simulink library "lib_accessory2"  (Simulink 4.1.1)
values from neighbouring files (symbols this model uses):
  logFlag = 1    [advSACompMaskInit.m]    (also in advSACompMaskInitR13.m)
undefined symbols (not defined in the file or in its folder): acc_abc_dutycycle, acc_abc_init, acc_ac_dutycycle, acc_ac_init, acc_acdc_inverter_eff, acc_alt_init, acc_dcdc_eff, acc_ef_dutycycle, acc_ef_init, acc_elec_eff, acc_elec_efficiency, acc_elec_pwr, acc_mech_eff, acc_mech_pwr, acc_mech_trq, acc_op_dutycycle, acc_op_init, acc_ps_dutycycle, acc_ps_init, acc_sindafile, acc_wp_dutycycle, acc_wp_init, amb_tmp, ess_on, fc_on, generalName, map_spd, max_pwr, tc_gc_to_fc_ratio, time_step, vc_idle_bool, vc_idle_spd, vinf
libraries: lib_cosimulation x29, lib_accessory2 x15, lib_outputs x11, simulink3 x10, lib_accessory x8, lib_etc x2
(part 2 of 5)

== system lib_accessory2/Elec Aux Loads 14V Pwr/Engine ==
  Average Watts : Constant  Value=vinf.AuxLoads.Engine.AverageWatts
  Memory : Memory  X0=0  InheritSampleTime=off
      settings: RTWStateStorageClass=Auto
  On : Constant  Value=vinf.AuxLoads.Engine.On
  Product : Product  Inputs=4  Multiplication=Element-wise(.*)  SaturateOnIntegerOverflow=on
  Out1 : Outport  Port=1
  wires:
  Memory/1 -> Product/2
  [engine_on] -> Memory/1
  [key_on] -> Product/3
  On/1 -> Product/1
  Product/1 -> Out1/1
  Average Watts/1 -> Product/4

== system lib_accessory2/Elec Aux Loads 14V Pwr/ExternalLights ==
  Average Watts : Constant  Value=vinf.AuxLoads.ExternalLights.AverageWatts
  On : Constant  Value=vinf.AuxLoads.ExternalLights.On
  Product : Product  Inputs=3  Multiplication=Element-wise(.*)  SaturateOnIntegerOverflow=on
  Subsystem : lib_cosimulation/Subsystem  ModelName='ExternalLights'
  Out1 : Outport  Port=1
  wires:
  Average Watts/1 -> Product/3
  On/1 -> Product/1
  Subsystem/1 -> Product/2
  Product/1 -> Out1/1

== system lib_accessory2/Elec Aux Loads 14V Pwr/FrontHVAC ==
  Average Watts : Constant  Value=vinf.AuxLoads.FrontHVAC.AverageWatts
  On : Constant  Value=vinf.AuxLoads.FrontHVAC.On
  Product : Product  Inputs=3  Multiplication=Element-wise(.*)  SaturateOnIntegerOverflow=on
  Subsystem : lib_cosimulation/Subsystem  ModelName='FrontHVAC'
  Out1 : Outport  Port=1
  wires:
  Average Watts/1 -> Product/3
  On/1 -> Product/1
  Subsystem/1 -> Product/2
  Product/1 -> Out1/1

== system lib_accessory2/Elec Aux Loads 14V Pwr/FrontWipers ==
  Average Watts : Constant  Value=vinf.AuxLoads.FrontWipers.AverageWatts
  On : Constant  Value=vinf.AuxLoads.FrontWipers.On
  Product : Product  Inputs=3  Multiplication=Element-wise(.*)  SaturateOnIntegerOverflow=on
  Subsystem : lib_cosimulation/Subsystem  ModelName='FrontWipers'
  Out1 : Outport  Port=1
  wires:
  Average Watts/1 -> Product/3
  On/1 -> Product/1
  Subsystem/1 -> Product/2
  Product/1 -> Out1/1

== system lib_accessory2/Elec Aux Loads 14V Pwr/HeatedSeats ==
  Average Watts : Constant  Value=vinf.AuxLoads.HeatedSeats.AverageWatts
  Num : Constant  Value=vinf.AuxLoads.HeatedSeats.Num
  On : Constant  Value=vinf.AuxLoads.HeatedSeats.On
  Product : Product  Inputs=4  Multiplication=Element-wise(.*)  SaturateOnIntegerOverflow=on
  Subsystem : lib_cosimulation/Subsystem  ModelName='HeatedSeats'
  Out1 : Outport  Port=1
  wires:
  Subsystem/1 -> Product/3
  Product/1 -> Out1/1
  Average Watts/1 -> Product/4
  On/1 -> Product/1
  Num/1 -> Product/2

== system lib_accessory2/Elec Aux Loads 14V Pwr/Misc ==
  Average Watts : Constant  Value=vinf.AuxLoads.Misc.AverageWatts
  On : Constant  Value=vinf.AuxLoads.Misc.On
  Product : Product  Inputs=3  Multiplication=Element-wise(.*)  SaturateOnIntegerOverflow=on
  Out1 : Outport  Port=1
  wires:
  Average Watts/1 -> Product/3
  [key_on] -> Product/2
  On/1 -> Product/1
  Product/1 -> Out1/1

== system lib_accessory2/Elec Aux Loads 14V Pwr/RadiatorCoolingFan ==
  Average Watts : Constant  Value=vinf.AuxLoads.RadiatorCoolingFan.AverageWatts
  On : Constant  Value=vinf.AuxLoads.RadiatorCoolingFan.On
  Product : Product  Inputs=3  Multiplication=Element-wise(.*)  SaturateOnIntegerOverflow=on
  Subsystem : lib_cosimulation/Subsystem  ModelName='RadiatorCoolingFan'
  Out1 : Outport  Port=1
  wires:
  Average Watts/1 -> Product/3
  On/1 -> Product/1
  Subsystem/1 -> Product/2
  Product/1 -> Out1/1

== system lib_accessory2/Elec Aux Loads 14V Pwr/Radio ==
  Average Watts : Constant  Value=vinf.AuxLoads.Radio.AverageWatts
  Num : Constant  Value=vinf.AuxLoads.Radio.Num
  On : Constant  Value=vinf.AuxLoads.Radio.On
  Product : Product  Inputs=4  Multiplication=Element-wise(.*)  SaturateOnIntegerOverflow=on
  Subsystem : lib_cosimulation/Subsystem  ModelName='Radio'
  Out1 : Outport  Port=1
  wires:
  Subsystem/1 -> Product/3
  Average Watts/1 -> Product/4
  On/1 -> Product/1
  Num/1 -> Product/2
  Product/1 -> Out1/1

== system lib_accessory2/Elec Aux Loads 14V Pwr/RearDefrost ==
  Average Watts : Constant  Value=vinf.AuxLoads.RearDefrost.AverageWatts
  On : Constant  Value=vinf.AuxLoads.RearDefrost.On
  Product : Product  Inputs=3  Multiplication=Element-wise(.*)  SaturateOnIntegerOverflow=on
  Subsystem : lib_cosimulation/Subsystem  ModelName='RearDefrost'
  Out1 : Outport  Port=1
  wires:
  Subsystem/1 -> Product/2
  Average Watts/1 -> Product/3
  On/1 -> Product/1
  Product/1 -> Out1/1

== system lib_accessory2/Elec Aux Loads 14V Pwr/RearHVAC ==
  Average Watts : Constant  Value=vinf.AuxLoads.RearHVAC.AverageWatts
  On : Constant  Value=vinf.AuxLoads.RearHVAC.On
  Product : Product  Inputs=3  Multiplication=Element-wise(.*)  SaturateOnIntegerOverflow=on
  Subsystem : lib_cosimulation/Subsystem  ModelName='RearHVAC'
  Out1 : Outport  Port=1
  wires:
  Average Watts/1 -> Product/3
  On/1 -> Product/1
  Subsystem/1 -> Product/2
  Product/1 -> Out1/1

== system lib_accessory2/Elec Aux Loads 14V Pwr/RearWipers ==
  Average Watts : Constant  Value=vinf.AuxLoads.RearWipers.AverageWatts
  On : Constant  Value=vinf.AuxLoads.RearWipers.On
  Product : Product  Inputs=3  Multiplication=Element-wise(.*)  SaturateOnIntegerOverflow=on
  Subsystem : lib_cosimulation/Subsystem  ModelName='RearWipers'
  Out1 : Outport  Port=1
  wires:
  Average Watts/1 -> Product/3
  On/1 -> Product/1
  Subsystem/1 -> Product/2
  Product/1 -> Out1/1

== system lib_accessory2/Elec Aux Loads 14V Pwr/Starter ==
  Product1 : Product  Inputs=2  Multiplication=Element-wise(.*)  SaturateOnIntegerOverflow=on
  Starter : lib_cosimulation/14V Load Control/Starter
      settings: RTWFcnNameOpts=Auto  RTWFileNameOpts=Auto
  starter_load (power) : Constant  Value=vinf.AuxLoads.Starter.AverageWatts
  Out1 : Outport  Port=1
  wires:
  Starter/1 -> Product1/1
  starter_load (power)/1 -> Product1/2
  Product1/1 -> Out1/1

== system lib_accessory2/Elec Aux Loads 14V Pwr/TurnSignals ==
  Average Watts : Constant  Value=vinf.AuxLoads.TurnSignals.AverageWatts
  On : Constant  Value=vinf.AuxLoads.TurnSignals.On
  Product : Product  Inputs=3  Multiplication=Element-wise(.*)  SaturateOnIntegerOverflow=on
  Subsystem : lib_cosimulation/Subsystem  ModelName='TurnSignals'
  Out1 : Outport  Port=1
  wires:
  Average Watts/1 -> Product/3
  On/1 -> Product/1
  Subsystem/1 -> Product/2
  Product/1 -> Out1/1

== system lib_accessory2/Elec Aux Loads HiV Pwr/CurrentLoad1 ==
  Average Watts : Constant  Value=vinf.AuxLoads.CurrentLoad1.AverageWatts
  On : Constant  Value=vinf.AuxLoads.CurrentLoad1.On
  Product : Product  Inputs=3  Multiplication=Element-wise(.*)  SaturateOnIntegerOverflow=on
  Subsystem : lib_cosimulation/Subsystem  ModelName='CurrentLoad1'
  Out1 : Outport  Port=1
  wires:
  Product/1 -> Out1/1
  Subsystem/1 -> Product/2
  On/1 -> Product/1
  Average Watts/1 -> Product/3

== system lib_accessory2/Elec Aux Loads HiV Pwr/PowerLoad1 ==
  Average Watts : Constant  Value=vinf.AuxLoads.PowerLoad1.AverageWatts
  On : Constant  Value=vinf.AuxLoads.PowerLoad1.On
  Product : Product  Inputs=3  Multiplication=Element-wise(.*)  SaturateOnIntegerOverflow=on
  Subsystem : lib_cosimulation/Subsystem  ModelName='PowerLoad1'
  Out1 : Outport  Port=1
  wires:
  Product/1 -> Out1/1
  On/1 -> Product/1
  Average Watts/1 -> Product/3
  Subsystem/1 -> Product/2

== system lib_accessory2/Elec Aux Loads HiV Pwr/PowerLoad2 ==
  Average Watts : Constant  Value=vinf.AuxLoads.PowerLoad2.AverageWatts
  On : Constant  Value=vinf.AuxLoads.PowerLoad2.On
  Product : Product  Inputs=3  Multiplication=Element-wise(.*)  SaturateOnIntegerOverflow=on
  Subsystem : lib_cosimulation/Subsystem  ModelName='PowerLoad2'
  Out1 : Outport  Port=1
  wires:
  Subsystem/1 -> Product/2
  Average Watts/1 -> Product/3
  On/1 -> Product/1
  Product/1 -> Out1/1

== system lib_accessory2/Elec Aux Loads HiV Pwr/PowerLoad3 ==
  Average Watts : Constant  Value=vinf.AuxLoads.PowerLoad3.AverageWatts
  On : Constant  Value=vinf.AuxLoads.PowerLoad3.On
  Product : Product  Inputs=3  Multiplication=Element-wise(.*)  SaturateOnIntegerOverflow=on
  Subsystem : lib_cosimulation/Subsystem  ModelName='PowerLoad3'
  Out1 : Outport  Port=1
  wires:
  Product/1 -> Out1/1
  On/1 -> Product/1
  Average Watts/1 -> Product/3
  Subsystem/1 -> Product/2

== system lib_accessory2/Elec Aux Loads HiV Pwr/SpeedLoad1 ==
  On : Constant  Value=vinf.AuxLoads.SpeedLoad1.On
  Product : Product  Inputs=3  Multiplication=Element-wise(.*)  SaturateOnIntegerOverflow=on
  Subsystem : lib_cosimulation/Subsystem  ModelName='SpeedLoad1'
  "rad/s -> rpm1" : Gain  Gain=60/(2*pi)  Multiplication=Element-wise(K.*u)  SaturateOnIntegerOverflow=on
  speed (rpm) vs load (watts) : Lookup  InputValues=[vinf.AuxLoads.SpeedLoad1.Data(1,1),vinf.AuxLoads.SpeedLoad1.Data(2,1)]  OutputValues=[vinf.AuxLoads.SpeedLoad1.Data(1,2),vinf.AuxLoads.SpeedLoad1.Data(2,2)]
  Out1 : Outport  Port=1
  wires:
  Product/1 -> Out1/1
  Subsystem/1 -> Product/2
  On/1 -> Product/1
  speed (rpm) vs load (watts)/1 -> Product/3
  [w_APU_speed] -> "rad/s -> rpm1"/1
  "rad/s -> rpm1"/1 -> speed (rpm) vs load (watts)/1

== system lib_accessory2/Elec Aux Loads HiV Pwr/Starter ==
  Product1 : Product  Inputs=2  Multiplication=Element-wise(.*)  SaturateOnIntegerOverflow=on
  Starter : Subsystem
      settings: RTWFcnNameOpts=Auto  RTWFileNameOpts=Auto
  starter_load (power) : Constant  Value=vinf.AuxLoads.Starter.AverageWatts
  Out1 : Outport  Port=1
  wires:
  Product1/1 -> Out1/1
  starter_load (power)/1 -> Product1/2
  Starter/1(Starter_OnOff_Control) -> Product1/1

== system lib_accessory2/SubLibraries/Shaft Speed and Actual Load Auxiliary Device ==
  angular  speed of engine  shaft (rad/s) : Inport  Port=1  LatchInput=off
  load on device (W) : Inport  Port=2  LatchInput=off
  Gain : Gain  Gain=1/conv_eff  Multiplication=Element-wise(K.*u)  SaturateOnIntegerOverflow=on
  Mux : Mux  Inputs=2
  device power requirements : MATLABFcn  MATLABFcn=feval(pwr_func, u(1), u(2))  OutputDimensions=1  OutputSignalType=real  Output1D=on
  powr required by device (W) : Outport  Port=1
  wires:
  angular  speed of engine  shaft (rad/s)/1 -> Mux/1
  Gain/1 -> Mux/2
  load on device (W)/1 -> Gain/1
  device power requirements/1 -> powr required by device (W)/1
  Mux/1 -> device power requirements/1

== system lib_accessory2/SubLibraries/Shaft Speed and Actual Load Auxiliary Device--lookuptable ==
  angular  speed of engine  shaft (rad/s) : Inport  Port=1  LatchInput=off
  load on device (W) : Inport  Port=2  LatchInput=off
  Constant : Constant  Value=0.0
  Constant1 : Constant  Value=eps
  Gain : Gain  Gain=1/conv_eff  Multiplication=Element-wise(K.*u)  SaturateOnIntegerOverflow=on
  Look-Up Table : Lookup  InputValues=map_spd  OutputValues=max_pwr
  Look-Up Table (2-D) : simulink3/Functions & Tables/Look-Up Table (2-D)  x=map_spd  y=map_load  t=pwr_map
  Product : Product  Inputs=*/  Multiplication=Element-wise(.*)  SaturateOnIntegerOverflow=on
  Relational Operator : RelationalOperator  Operator=~=
  Saturation : Saturate  UpperLimit=1.0  LowerLimit=0.0  LinearizeAsGain=on
  Saturation1 : Saturate  UpperLimit=maxSpd  LowerLimit=minSpd  LinearizeAsGain=on
  Switch : Switch  Threshold=0.5
  powr required by device (W) : Outport  Port=1
  wires:
  load on device (W)/1 -> Gain/1
  Look-Up Table (2-D)/1 -> powr required by device (W)/1
  angular  speed of engine  shaft (rad/s)/1 -> Saturation1/1
  [spd] -> Look-Up Table (2-D)/1
  Saturation1/1 -> [spd]
  Gain/1 -> Product/1
  [spd] -> Look-Up Table/1
  Product/1 -> Saturation/1
  Saturation/1 -> Look-Up Table (2-D)/2
  Look-Up Table/1 -> Relational Operator/1, Switch/1
  Constant/1 -> Relational Operator/2
  Relational Operator/1 -> Switch/2
  Constant1/1 -> Switch/3
  Switch/1 -> Product/2

== system lib_accessory2/SubLibraries/Shaft Speed and Time Loaded Auxiliary Device ==
  angular  speed of engine  shaft (rad/s) : Inport  Port=1  LatchInput=off
  elapsed time since start of simulation (s) : Inport  Port=2  LatchInput=off
  Mux : Mux  Inputs=2
  Sat : Saturate  UpperLimit=1.0  LowerLimit=0.0  LinearizeAsGain=on
  device duty  schedule by time : Subsystem  mask(Repeating table){t=acc_duty(:,1), y=acc_duty(:,2)}
      mask prompts: t "Input values:"; y "Output values:"
      mask help:
      | Repeating table.
      | Enter values of input and output for first cycle.
      mask init:
      | period = max(@1);
      settings: RTWFcnNameOpts=Auto  RTWFileNameOpts=Auto
      mask Help: Repeats cycle given in table. Input values should be monotonically increasing.
  device power requirements : MATLABFcn  MATLABFcn=feval(pwr_func, u(1), u(2))  OutputDimensions=1  OutputSignalType=real  Output1D=on
  powr required by device (W) : Outport  Port=1
  "duty cycle (1=\"on full power\" & 0=\"off\")" : Outport  Port=2
  wires:
  Mux/1 -> device power requirements/1
  angular  speed of engine  shaft (rad/s)/1 -> Mux/1
  device power requirements/1 -> powr required by device (W)/1
  elapsed time since start of simulation (s)/1 -> device duty  schedule by time/1(distance travelled (m))
  device duty  schedule by time/1(out_1) -> Sat/1
  Sat/1 -> Mux/2, "duty cycle (1=\"on full power\" & 0=\"off\")"/1

== system lib_accessory2/SubLibraries/Shaft Speed and Time Loaded Auxiliary Device--lookuptable ==
  angular  speed of engine  shaft (rad/s) : Inport  Port=1  LatchInput=off
  elapsed time since start of simulation (s) : Inport  Port=2  LatchInput=off
  Look-Up Table (2-D) : simulink3/Functions & Tables/Look-Up Table (2-D)  x=map_spd  y=map_load  t=pwr_map
  Sat : Saturate  UpperLimit=1.0  LowerLimit=0.0  LinearizeAsGain=on
  Sat1 : Saturate  UpperLimit=maxSpd  LowerLimit=minSpd  LinearizeAsGain=on
  device duty  schedule by time : Subsystem  mask(Repeating table){t=acc_duty(:,1), y=acc_duty(:,2)}
      mask prompts: t "Input values:"; y "Output values:"
      mask help:
      | Repeating table.
      | Enter values of input and output for first cycle.
      mask init:
      | period = max(@1);
      settings: RTWFcnNameOpts=Auto  RTWFileNameOpts=Auto
      mask Help: Repeats cycle given in table. Input values should be monotonically increasing.
  powr required by device (W) : Outport  Port=1
  "duty cycle (1=\"on full power\" & 0=\"off\")" : Outport  Port=2
  wires:
  Look-Up Table (2-D)/1 -> powr required by device (W)/1
  elapsed time since start of simulation (s)/1 -> device duty  schedule by time/1(distance travelled (m))
  device duty  schedule by time/1(out_1) -> Sat/1
  Sat/1 -> "duty cycle (1=\"on full power\" & 0=\"off\")"/1, Look-Up Table (2-D)/2
  angular  speed of engine  shaft (rad/s)/1 -> Sat1/1
  Sat1/1 -> Look-Up Table (2-D)/1

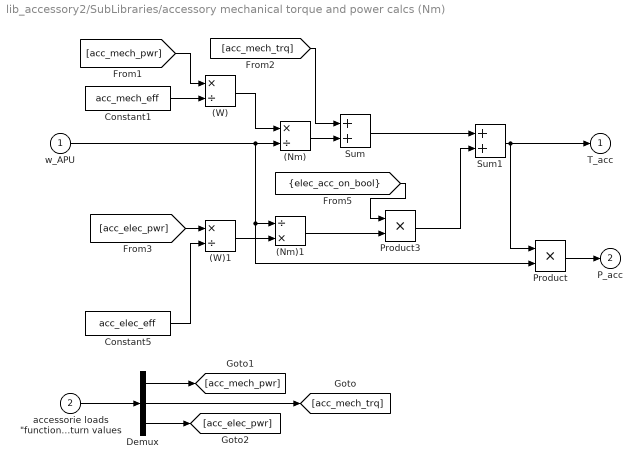
== system lib_accessory2/SubLibraries/accessory mechanical torque and power calcs (Nm) ==
  w_APU : Inport  Port=1  LatchInput=off
  "accessorie loads \"function\" return values" : Inport  Port=2  LatchInput=off
  (Nm) : Product  Inputs=*/  Multiplication=Element-wise(.*)  SaturateOnIntegerOverflow=on
  (Nm)1 : Product  Inputs=/*  Multiplication=Element-wise(.*)  SaturateOnIntegerOverflow=on
  (W) : Product  Inputs=*/  Multiplication=Element-wise(.*)  SaturateOnIntegerOverflow=on
  (W)1 : Product  Inputs=*/  Multiplication=Element-wise(.*)  SaturateOnIntegerOverflow=on
  Constant1 : Constant  Value=acc_mech_eff
  Constant5 : Constant  Value=acc_elec_eff
  Demux : Demux  Outputs=3  BusSelectionMode=off
  Product : Product  Inputs=2  Multiplication=Element-wise(.*)  SaturateOnIntegerOverflow=on
  Product3 : Product  Inputs=2  Multiplication=Element-wise(.*)  SaturateOnIntegerOverflow=on
  Sum : Sum  Inputs=++  SaturateOnIntegerOverflow=on
  Sum1 : Sum  Inputs=++  SaturateOnIntegerOverflow=on
  T_acc : Outport  Port=1  InitialOutput=0
  P_acc : Outport  Port=2  InitialOutput=0
  wires:
  "accessorie loads \"function\" return values"/1 -> Demux/1
  Demux/3 -> [acc_elec_pwr]
  Demux/1 -> [acc_mech_pwr]
  Demux/2 -> [acc_mech_trq]
  Product/1 -> P_acc/1
  (W)/1 -> (Nm)/1
  Constant1/1 -> (W)/2
  [acc_mech_pwr] -> (W)/1
  (Nm)/1 -> Sum/2
  Sum/1 -> Sum1/1
  Sum1/1 -> Product/1, T_acc/1
  Constant5/1 -> (W)1/2
  (W)1/1 -> (Nm)1/2
  (Nm)1/1 -> Product3/2
  Product3/1 -> Sum1/2
  [elec_acc_on_bool] -> Product3/1
  [acc_mech_trq] -> Sum/1
  w_APU/1 -> (Nm)1/1, Product/2, (Nm)/2
  [acc_elec_pwr] -> (W)1/1

== system lib_accessory2/SubLibraries/data logging probes dummy ==
  In1 : Inport  Port=1  LatchInput=off
  Terminator : Terminator
  wires:
  In1/1 -> Terminator/1

== system lib_accessory2/SubLibraries/data logging probes for conventional mechanical loads ==
  In1 : Inport  Port=1  LatchInput=off
  Demux : Demux  Outputs=12  BusSelectionMode=off
  To Workspace : ToWorkspace  VariableName=acc_ac_pwr_out_a  SampleTime=-1  SaveFormat=Array
  To Workspace1 : ToWorkspace  VariableName=acc_pwr_steer_pwr_out_a  SampleTime=-1  SaveFormat=Array
  To Workspace10 : ToWorkspace  VariableName=acc_op_pwr_out_a  SampleTime=-1  SaveFormat=Array
  To Workspace11 : ToWorkspace  VariableName=acc_op_duty  SampleTime=-1  SaveFormat=Array
  To Workspace2 : ToWorkspace  VariableName=acc_air_comp_pwr_out_a  SampleTime=-1  SaveFormat=Array
  To Workspace3 : ToWorkspace  VariableName=acc_eng_fan_pwr_out_a  SampleTime=-1  SaveFormat=Array
  To Workspace4 : ToWorkspace  VariableName=acc_alt_pwr_out_a  SampleTime=-1  SaveFormat=Array
  To Workspace5 : ToWorkspace  VariableName=acc_14elec_pwr_out_a  SampleTime=-1  SaveFormat=Array
  To Workspace6 : ToWorkspace  VariableName=acc_ps_duty  SampleTime=-1  SaveFormat=Array
  To Workspace7 : ToWorkspace  VariableName=acc_air_comp_duty  SampleTime=-1  SaveFormat=Array
  To Workspace8 : ToWorkspace  VariableName=acc_fan_duty  SampleTime=-1  SaveFormat=Array
  To Workspace9 : ToWorkspace  VariableName=acc_ac_duty  SampleTime=-1  SaveFormat=Array
  wires:
  Demux/12 -> To Workspace11/1
  Demux/11 -> To Workspace10/1
  Demux/10 -> To Workspace9/1
  Demux/9 -> To Workspace8/1
  Demux/8 -> To Workspace7/1
  Demux/7 -> To Workspace6/1
  Demux/6 -> To Workspace5/1
  Demux/5 -> To Workspace4/1
  Demux/4 -> To Workspace3/1
  Demux/3 -> To Workspace2/1
  Demux/2 -> To Workspace1/1
  Demux/1 -> To Workspace/1
  In1/1 -> Demux/1

== system lib_accessory2/SubLibraries/data probes ==
  In1 : Inport  Port=1  LatchInput=off
  data logging probes for conventional mechanical loads : lib_accessory/SubLibraries/data logging probes for conventional mechanical loads
      settings: RTWFcnNameOpts=Auto  RTWFileNameOpts=Auto
  wires:
  In1/1 -> data logging probes for conventional mechanical loads/1

== system lib_accessory2/SubLibraries/electrical power logging ==
  In1 : Inport  Port=1  LatchInput=off
  Gain : Gain  Gain=acc_elec_eff  Multiplication=Element-wise(K.*u)  SaturateOnIntegerOverflow=on
  enhancedToWorkspace : Subsystem  TreatAsAtomicUnit=on  mask(enhancedToWorkspace){generalName=generalName, specificName=elec_pwr_out_a, logFlag=logFlag}
      mask prompts: generalName "General Name [char-evaluated]"; specificName "Specific Name [char-literal]"; logFlag "Enable flag (1=on,0=off)"
      mask help: A wrapper for the Simulink "To Workspace" block that allows you to evaluate the name of the variable to log to workspace. This is useful to avoid the double logging errors that occur when you pull in two library models that attempt to log to the same variable.
      mask init:
      | enhancedToWsMaker
      settings: CopyFcn=breakLinkCopyFcn  ParentCloseFcn=breakLinkParCloseFcn  RTWFcnNameOpts=Auto  RTWFileNameOpts=Auto
      mask Help:
      | <h2>Enhanced To Workspace Block</h2>
      | <h3>Parameters</h3>
      | <UL>
      | <li><b>General Name:</b> This is the more general name of the variable. Variables are saved to the workspace as <i>generalName_specificName</i>. Note that this is an evaluated variable. If you would like to type in the value directly, it must be surrounded with single quotes. Otherwise you can input the name of a variable containing a char string.</li>
      | <li><b>Specific Name:</b> This is the specific name of the variable. Note that this is input as a char literal (i.e., you don't need quotes).</li>
      | <li><b>Enable Flag:</b> This flag should have the value of 0 or 1. If 0, the variable will not be logged to the workspace. If 1, the variable will be logged. This is done so that variable logging can be turned off to improve speed.</li>
      | </ul>
      | <h3>Overview</h3>
      | <p>The enhanced to workspace block was put together to allow one to dynamically resolve variable names at run time in simulink. This is most powerful when used in conjunction with a masked subsystem to allow multiple instances of that masked subsytem to be used in the same model. The strategy is to set the generalName in the block mask which will allow the block to change the general name for all variable logging on the fly.
      | <h3>Helper Files</h3>
      | <p>Three m-files are required by the enhancedToWorkspace block. These files are located in the &lt; ADVISOR root &gt;/GUI directory :
      | <ul>
      | <li><i>enhancedToWsMaker.m</i> This file runs the mask initialization for the block</li>
      | <li><i>breakLinkCopyFcn.m</i> This file is used by the block callback when the simulink block is copied. It is necessary to break the link to the enhancedToWorkspace similar to the To Workspace block in order for it to be able to configure itself. (Try copying simulink's To Workspace block--it is impossible to make a link)</li>
      | <li><i>breakLinkParCloseFcn.m</i> This file is similar to the breakLinkCopyFcn and is used when a parent system is closed</li>
      | </ul>
      | <hr>
      | 
      | <p>Created 2003-Jan-21, Michael Patrick O'Keefe, NREL</p>
      | 
      | <!--
      | <VARDEF>
      | <H3>var_name</H3>
      | <UL>
      | <LI><B>data type</B> data type here</LI>
      | <LI><B>units</B> units here</LI>
      | <LI><B>vehicle type</B> vehicle type here</LI>
      | <LI><B>description</B> description here</LI>
      | </UL>
      | </VARDEF>
      | -->
      mask Display: disp([generalName,'_',specificName])
  enhancedToWorkspace1 : Subsystem  TreatAsAtomicUnit=on  mask(enhancedToWorkspace){generalName=generalName, specificName=elec_pwr_in_a, logFlag=logFlag}
      mask prompts: generalName "General Name [char-evaluated]"; specificName "Specific Name [char-literal]"; logFlag "Enable flag (1=on,0=off)"
      mask help: A wrapper for the Simulink "To Workspace" block that allows you to evaluate the name of the variable to log to workspace. This is useful to avoid the double logging errors that occur when you pull in two library models that attempt to log to the same variable.
      mask init:
      | enhancedToWsMaker
      settings: CopyFcn=breakLinkCopyFcn  ParentCloseFcn=breakLinkParCloseFcn  RTWFcnNameOpts=Auto  RTWFileNameOpts=Auto
      mask Help:
      | <h2>Enhanced To Workspace Block</h2>
      | <h3>Parameters</h3>
      | <UL>
      | <li><b>General Name:</b> This is the more general name of the variable. Variables are saved to the workspace as <i>generalName_specificName</i>. Note that this is an evaluated variable. If you would like to type in the value directly, it must be surrounded with single quotes. Otherwise you can input the name of a variable containing a char string.</li>
      | <li><b>Specific Name:</b> This is the specific name of the variable. Note that this is input as a char literal (i.e., you don't need quotes).</li>
      | <li><b>Enable Flag:</b> This flag should have the value of 0 or 1. If 0, the variable will not be logged to the workspace. If 1, the variable will be logged. This is done so that variable logging can be turned off to improve speed.</li>
      | </ul>
      | <h3>Overview</h3>
      | <p>The enhanced to workspace block was put together to allow one to dynamically resolve variable names at run time in simulink. This is most powerful when used in conjunction with a masked subsystem to allow multiple instances of that masked subsytem to be used in the same model. The strategy is to set the generalName in the block mask which will allow the block to change the general name for all variable logging on the fly.
      | <h3>Helper Files</h3>
      | <p>Three m-files are required by the enhancedToWorkspace block. These files are located in the &lt; ADVISOR root &gt;/GUI directory :
      | <ul>
      | <li><i>enhancedToWsMaker.m</i> This file runs the mask initialization for the block</li>
      | <li><i>breakLinkCopyFcn.m</i> This file is used by the block callback when the simulink block is copied. It is necessary to break the link to the enhancedToWorkspace similar to the To Workspace block in order for it to be able to configure itself. (Try copying simulink's To Workspace block--it is impossible to make a link)</li>
      | <li><i>breakLinkParCloseFcn.m</i> This file is similar to the breakLinkCopyFcn and is used when a parent system is closed</li>
      | </ul>
      | <hr>
      | 
      | <p>Created 2003-Jan-21, Michael Patrick O'Keefe, NREL</p>
      | 
      | <!--
      | <VARDEF>
      | <H3>var_name</H3>
      | <UL>
      | <LI><B>data type</B> data type here</LI>
      | <LI><B>units</B> units here</LI>
      | <LI><B>vehicle type</B> vehicle type here</LI>
      | <LI><B>description</B> description here</LI>
      | </UL>
      | </VARDEF>
      | -->
      mask Display: disp([generalName,'_',specificName])
  wires:
  In1/1 -> Gain/1, enhancedToWorkspace1/1(In1)
  Gain/1 -> enhancedToWorkspace/1(In1)

== system lib_accessory2/SubLibraries/mechanical power logging ==
  In1 : Inport  Port=1  LatchInput=off
  Gain : Gain  Gain=acc_mech_eff  Multiplication=Element-wise(K.*u)  SaturateOnIntegerOverflow=on
  f : Subsystem  TreatAsAtomicUnit=on  mask(enhancedToWorkspace){generalName=generalName, specificName=mech_pwr_out_a, logFlag=logFlag}
      mask prompts: generalName "General Name [char-evaluated]"; specificName "Specific Name [char-literal]"; logFlag "Enable flag (1=on,0=off)"
      mask help: A wrapper for the Simulink "To Workspace" block that allows you to evaluate the name of the variable to log to workspace. This is useful to avoid the double logging errors that occur when you pull in two library models that attempt to log to the same variable.
      mask init:
      | enhancedToWsMaker
      settings: CopyFcn=breakLinkCopyFcn  ParentCloseFcn=breakLinkParCloseFcn  RTWFcnNameOpts=Auto  RTWFileNameOpts=Auto
      mask Help:
      | <h2>Enhanced To Workspace Block</h2>
      | <h3>Parameters</h3>
      | <UL>
      | <li><b>General Name:</b> This is the more general name of the variable. Variables are saved to the workspace as <i>generalName_specificName</i>. Note that this is an evaluated variable. If you would like to type in the value directly, it must be surrounded with single quotes. Otherwise you can input the name of a variable containing a char string.</li>
      | <li><b>Specific Name:</b> This is the specific name of the variable. Note that this is input as a char literal (i.e., you don't need quotes).</li>
      | <li><b>Enable Flag:</b> This flag should have the value of 0 or 1. If 0, the variable will not be logged to the workspace. If 1, the variable will be logged. This is done so that variable logging can be turned off to improve speed.</li>
      | </ul>
      | <h3>Overview</h3>
      | <p>The enhanced to workspace block was put together to allow one to dynamically resolve variable names at run time in simulink. This is most powerful when used in conjunction with a masked subsystem to allow multiple instances of that masked subsytem to be used in the same model. The strategy is to set the generalName in the block mask which will allow the block to change the general name for all variable logging on the fly.
      | <h3>Helper Files</h3>
      | <p>Three m-files are required by the enhancedToWorkspace block. These files are located in the &lt; ADVISOR root &gt;/GUI directory :
      | <ul>
      | <li><i>enhancedToWsMaker.m</i> This file runs the mask initialization for the block</li>
      | <li><i>breakLinkCopyFcn.m</i> This file is used by the block callback when the simulink block is copied. It is necessary to break the link to the enhancedToWorkspace similar to the To Workspace block in order for it to be able to configure itself. (Try copying simulink's To Workspace block--it is impossible to make a link)</li>
      | <li><i>breakLinkParCloseFcn.m</i> This file is similar to the breakLinkCopyFcn and is used when a parent system is closed</li>
      | </ul>
      | <hr>
      | 
      | <p>Created 2003-Jan-21, Michael Patrick O'Keefe, NREL</p>
      | 
      | <!--
      | <VARDEF>
      | <H3>var_name</H3>
      | <UL>
      | <LI><B>data type</B> data type here</LI>
      | <LI><B>units</B> units here</LI>
      | <LI><B>vehicle type</B> vehicle type here</LI>
      | <LI><B>description</B> description here</LI>
      | </UL>
      | </VARDEF>
      | -->
      mask Display: disp([generalName,'_',specificName])
  f1 : Subsystem  TreatAsAtomicUnit=on  mask(enhancedToWorkspace){generalName=generalName, specificName=mech_pwr_in_a, logFlag=logFlag}
      mask prompts: generalName "General Name [char-evaluated]"; specificName "Specific Name [char-literal]"; logFlag "Enable flag (1=on,0=off)"
      mask help: A wrapper for the Simulink "To Workspace" block that allows you to evaluate the name of the variable to log to workspace. This is useful to avoid the double logging errors that occur when you pull in two library models that attempt to log to the same variable.
      mask init:
      | enhancedToWsMaker
      settings: CopyFcn=breakLinkCopyFcn  ParentCloseFcn=breakLinkParCloseFcn  RTWFcnNameOpts=Auto  RTWFileNameOpts=Auto
      mask Help:
      | <h2>Enhanced To Workspace Block</h2>
      | <h3>Parameters</h3>
      | <UL>
      | <li><b>General Name:</b> This is the more general name of the variable. Variables are saved to the workspace as <i>generalName_specificName</i>. Note that this is an evaluated variable. If you would like to type in the value directly, it must be surrounded with single quotes. Otherwise you can input the name of a variable containing a char string.</li>
      | <li><b>Specific Name:</b> This is the specific name of the variable. Note that this is input as a char literal (i.e., you don't need quotes).</li>
      | <li><b>Enable Flag:</b> This flag should have the value of 0 or 1. If 0, the variable will not be logged to the workspace. If 1, the variable will be logged. This is done so that variable logging can be turned off to improve speed.</li>
      | </ul>
      | <h3>Overview</h3>
      | <p>The enhanced to workspace block was put together to allow one to dynamically resolve variable names at run time in simulink. This is most powerful when used in conjunction with a masked subsystem to allow multiple instances of that masked subsytem to be used in the same model. The strategy is to set the generalName in the block mask which will allow the block to change the general name for all variable logging on the fly.
      | <h3>Helper Files</h3>
      | <p>Three m-files are required by the enhancedToWorkspace block. These files are located in the &lt; ADVISOR root &gt;/GUI directory :
      | <ul>
      | <li><i>enhancedToWsMaker.m</i> This file runs the mask initialization for the block</li>
      | <li><i>breakLinkCopyFcn.m</i> This file is used by the block callback when the simulink block is copied. It is necessary to break the link to the enhancedToWorkspace similar to the To Workspace block in order for it to be able to configure itself. (Try copying simulink's To Workspace block--it is impossible to make a link)</li>
      | <li><i>breakLinkParCloseFcn.m</i> This file is similar to the breakLinkCopyFcn and is used when a parent system is closed</li>
      | </ul>
      | <hr>
      | 
      | <p>Created 2003-Jan-21, Michael Patrick O'Keefe, NREL</p>
      | 
      | <!--
      | <VARDEF>
      | <H3>var_name</H3>
      | <UL>
      | <LI><B>data type</B> data type here</LI>
      | <LI><B>units</B> units here</LI>
      | <LI><B>vehicle type</B> vehicle type here</LI>
      | <LI><B>description</B> description here</LI>
      | </UL>
      | </VARDEF>
      | -->
      mask Display: disp([generalName,'_',specificName])
  wires:
  In1/1 -> Gain/1, f1/1(In1)
  Gain/1 -> f/1(In1)
